simulink model "Dref_fixedstep"  (R2021a)
settings: Solver=ode23t  StartTime=0.0  StopTime=2  FixedStep=1e-6  RelTol=1e-3
libraries: spsSeriesRLCBranchLib x7, spsDiodeLib x5, spsMosfetLib x2, spsCurrentMeasurementLib x1, spsPVArrayLib x1, simulink x1, spsVoltageMeasurementLib x1, spspowerguiLib x1
settings Model: Creator=Kryptic  LastModifiedBy=Kryptic

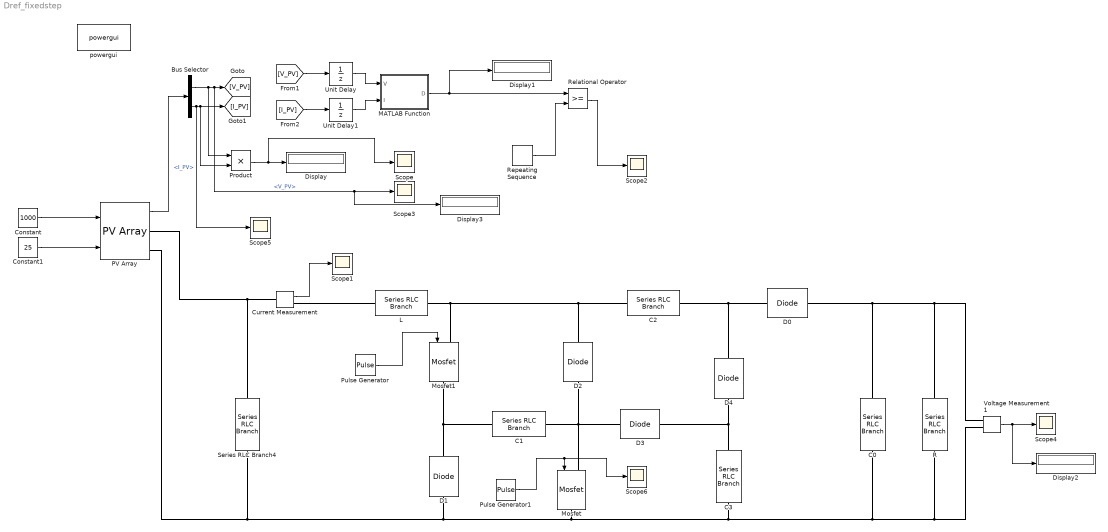
== system Dref_fixedstep ==
  Bus Selector : BusSelector  OutputSignals=V_PV,I_PV
  C0 : spsSeriesRLCBranchLib/Series RLC Branch  LConnTagsString=__new0  RConnTagsString=__new0  BranchType=C  Resistance=1  Inductance=1e-3  SetiL0=off  InitialCurrent=0  Capacitance=1e-4  Setx0=off  InitialVoltage=0  Measurements=None
  C1 : spsSeriesRLCBranchLib/Series RLC Branch  LConnTagsString=__new0  RConnTagsString=__new0  BranchType=C  Resistance=1  Inductance=1e-3  SetiL0=off  InitialCurrent=0  Capacitance=8.2e-6  Setx0=off  InitialVoltage=0  Measurements=None
  C2 : spsSeriesRLCBranchLib/Series RLC Branch  LConnTagsString=__new0  RConnTagsString=__new0  BranchType=C  Resistance=1  Inductance=1e-3  SetiL0=off  InitialCurrent=0  Capacitance=.62e-6  Setx0=off  InitialVoltage=0  Measurements=None
  C3 : spsSeriesRLCBranchLib/Series RLC Branch  LConnTagsString=__new0  RConnTagsString=__new0  BranchType=C  Resistance=1  Inductance=1e-3  SetiL0=off  InitialCurrent=0  Capacitance=1.3e-6  Setx0=off  InitialVoltage=0  Measurements=None
  Constant : Constant  Value=1000
  Constant1 : Constant  Value=25
  Current Measurement : spsCurrentMeasurementLib/Current Measurement  PhasorSimulation=off  OutputType=Complex  PSBequivalent=0
  D0 : spsDiodeLib/Diode  Ron=0.001  Lon=0  Vf=1.50  IC=0  UseSnubber=0  Rs=500  Cs=250e-9  Measurements=off
  D1 : spsDiodeLib/Diode  Ron=0.001  Lon=0  Vf=0.86  IC=0  UseSnubber=0  Rs=500  Cs=250e-9  Measurements=off
  D2 : spsDiodeLib/Diode  Ron=0.001  Lon=0  Vf=0.86  IC=0  UseSnubber=0  Rs=500  Cs=250e-9  Measurements=off
  D3 : spsDiodeLib/Diode  Ron=0.001  Lon=0  Vf=0.86  IC=0  UseSnubber=0  Rs=500  Cs=250e-9  Measurements=off
  D4 : spsDiodeLib/Diode  Ron=0.001  Lon=0  Vf=1.50  IC=0  UseSnubber=0  Rs=500  Cs=250e-9  Measurements=off
  Display{,1..3} (4 alike) : Display
  L : spsSeriesRLCBranchLib/Series RLC Branch  LConnTagsString=__new0  RConnTagsString=__new0  BranchType=L  Resistance=1  Inductance=20e-3  SetiL0=off  InitialCurrent=0  Capacitance=1e-6  Setx0=off  InitialVoltage=0  Measurements=None
  MATLAB Function : MATLAB Function  TreatAsAtomicUnit=on
  Mosfet : spsMosfetLib/Mosfet  Ron=8.0e-3  Lon=0  Rd=0.01  Vfd=1.3  IC=0  Rs=1e5  Cs=inf  Measurements=off
  Mosfet1 : spsMosfetLib/Mosfet  Ron=8.0e-3  Lon=0  Rd=0.01  Vfd=1.3  IC=0  Rs=1e5  Cs=inf  Measurements=off
  PV Array : spsPVArrayLib/PV Array  Npar=1  Nser=1  PlotType=array @ 25 deg.C & specified irradiances  S_vec="[ 1000  500  100 ]"  Temp_C_vec="[ 45 25  ]"  ModuleName=User-defined  PlotWhenSelected=off  Pm=20.06  Ncell=60  Voc=21  Isc=1.2  Vm=17  Im=1.18  beta_Voc_pc=-.585  alpha_Isc_pc=.00367  beta_Voc=-0.12285  alpha_Isc=4.404e-05  IL=1.2439  I0=1.4121e-08  nI=0.7447  Rsh=22939.389  Rs=0.77008  RobustModel=off  RobustCellTemperature=313.3991  BAL=on  Tc=1e-6  Tfilter=5e-5
  Product : Product
  Pulse Generator : DiscretePulseGenerator  Period=30000  PulseWidth=11700
  Pulse Generator1 : DiscretePulseGenerator  Period=30000  PulseWidth=11700
  R : spsSeriesRLCBranchLib/Series RLC Branch  LConnTagsString=__new0  RConnTagsString=__new0  BranchType=R  Resistance=2645  Inductance=1e-3  SetiL0=off  InitialCurrent=0  Capacitance=1e-6  Setx0=off  InitialVoltage=0  Measurements=None
  Relational Operator : RelationalOperator  OutDataTypeStr=boolean  RndMeth=Simplest
  Repeating Sequence : simulink/Sources/Repeating Sequence  rep_seq_t=[0 1/30000]  rep_seq_y=[0 1]
  Scope{,1..6} (7 alike) : Scope
  Series RLC Branch4 : spsSeriesRLCBranchLib/Series RLC Branch  LConnTagsString=__new0  RConnTagsString=__new0  BranchType=RC  Resistance=0  Inductance=1e-3  SetiL0=off  InitialCurrent=0  Capacitance=2.2e-6  Setx0=off  InitialVoltage=0  Measurements=None
  Unit Delay : UnitDelay  SampleTime=-1  HasFrameUpgradeWarning=on
  Unit Delay1 : UnitDelay  SampleTime=-1  HasFrameUpgradeWarning=on
  Voltage Measurement1 : spsVoltageMeasurementLib/Voltage Measurement  PhasorSimulation=off  OutputType=Complex  PSBequivalent=0
  powergui : spspowerguiLib/powergui  Priority=1  SimulationMode=Discrete  SampleTime=1e-6  frequency=60  Iterations=50  frequencyindice=0  Pbase=100e6  ErrMax=1e-4  UnitsV=kV  UnitsW=MW  buscounter=0  FunctionMessages=off  echomessages=off  EnableUseOfTLC=off  CurrentSourceSwitches=off  DisableSnubberDevices=off  DisableRonSwitches=off  DisableVfSwitches=off  DisplayEquations=off  AutomaticDiscreteSolvers=off  SolverType=Tustin/Backward Euler (TBE)  Interpol=off  ExternalGateDelay=off  methode=off  Ts=100  x0status=blocks  SPID=on  SwTol=0  HookPort=off  NonlinearTolerance=1e-4  nMaxIteration=100  ContinueOnMaxIteration=off  RestoreLinks=warning  ResistiveCurrentMeasurement=off  Frange=[0:2:500]  Ylog=off  Xlog=on  ShowGrid=off  save=off  variable=ZData  structure=0  ZoomFFT=off  StartTime=0.0  cycles=1  DisplayStyle=1  fundamental=60  FreqAxis=off  MaxFrequency=1000  frequencyindicesteady=1  RmsSteady=1  display=off
  wires:
  MATLAB Function/1(D) -> Relational Operator/1, Display1/1
  Repeating Sequence/1 -> Relational Operator/2
  Product/1 -> Scope/1, Display/1
  [V_PV] -> Unit Delay/1
  [I_PV] -> Unit Delay1/1
  Relational Operator/1 -> Scope2/1
  Constant1/1 -> PV Array/2
  Constant/1 -> PV Array/1
  Bus Selector/2 -> Scope5/1, Product/2, [I_PV]  "<I_PV>"
  PV Array/1 -> Bus Selector/1
  Bus Selector/1 -> Product/1, Display3/1, Scope3/1, [V_PV]  "<V_PV>"
  Unit Delay1/1 -> MATLAB Function/2(I)
  Unit Delay/1 -> MATLAB Function/1(V)
  Voltage Measurement1/1 -> Scope4/1, Display2/1
  Pulse Generator/1 -> Mosfet1/1
  Pulse Generator1/1 -> Scope6/1, Mosfet/1
  Current Measurement/1 -> Scope1/1
  connections:
  D0/RConn1 -- C0/LConn1 -- R/LConn1 -- Voltage Measurement1/LConn1
  D1/LConn1 -- Mosfet1/RConn1 -- C1/LConn1
  C2/LConn1 -- D2/LConn1 -- L/RConn1 -- Mosfet1/LConn1
  D1/RConn1 -- Mosfet/RConn1 -- R/RConn1 -- Voltage Measurement1/LConn2 -- C0/RConn1 -- C3/RConn1 -- PV Array/RConn2 -- Series RLC Branch4/RConn1
  D3/RConn1 -- D4/LConn1 -- C3/LConn1
  D3/LConn1 -- C1/RConn1 -- D2/RConn1 -- Mosfet/LConn1
  D4/RConn1 -- C2/RConn1 -- D0/LConn1
  PV Array/RConn1 -- Series RLC Branch4/LConn1 -- Current Measurement/LConn1
  Current Measurement/RConn1 -- L/LConn1

== matlab function Dref_fixedstep/MATLAB Function ==
  data: V input; D output; I input
function D = DutyRatio(V, I)

Dmax = .95;
Dmin = 0;
Dinit = .95;
deltaD = .001;
persistent Vold Pold Dold;
dataType = 'double';
if isempty(Vold)
    Vold = 0;
    Pold = 0;
    Dold = Dinit;
end

P= V*I;
dV = V-Vold;
dP = P-Pold;

if dP ~= 0
    if dP<0
        if dV<0
            D = Dold - deltaD;
        else
            D = Dold + deltaD;
        end
    else
        if dV<0
            D = Dold + deltaD;
        else
            D = Dold - deltaD;
        end
    end
else D = Dold;
end

if D >= Dmax | D <= Dmin
    D = Dold;
end

Dold = D;
Vold = V;
Pold = P;
